simulink model "mintaveteles_FOXBORO_PI_szabalyozo"  (Simulink 8.7)
settings: Solver=VariableStepAuto  StartTime=0.0  StopTime=T_sim  RelTol=1e-3
values from neighbouring files (symbols this model uses):
  inv_u_stat = y_stat(i-1:end)    [Sebessegszabalyozas_sim.m]
  inv_y_stat = u_stat(i-1:end)    [Sebessegszabalyozas_sim.m]
  K = P1.Kp    [Sebessegszabalyozas_sim.m]
  K_C = 1/P1d.Numerator(2)*(1-exp(-Ts/T_cl))    [Sebessegszabalyozas_sim.m]
  P1d = c2d(sys,Ts,'zoh')    [Sebessegszabalyozas_sim.m]
  Ts = 0.01    [Sebessegszabalyozas_sim.m]
  u_sat = y_sat/K    [Sebessegszabalyozas_sim.m]
  u_stat = [0;100;200;250;300;350;400;450;500;550;600;700;750]    [Untitled.m]    (also in ident.mat = [0 100 200 300 400 500 600 700])
  y_stat = y_stat*K    [Sebessegszabalyozas_sim.m]    (also in Untitled.m = [0;  0;  0;  0; 42; 67; 80; 95;110;120;130;160;170]; ident.mat = [0 0 0 32 100 160 216 260])
  z_d = -P1d.Denominator(2)    [Sebessegszabalyozas_sim.m]
settings Model: Creator=Mester Ádám  LastModifiedBy=Mester Ádám
settings DataIOCC: LimitDataPoints=off  SaveFormat=Dataset
settings DebuggingCC: UnderspecifiedInitializationDetection=Simplified  MergeDetectMultiDrivingBlocksExec=error
settings HardwareCC: ProdBitPerPointer=64  ProdLargestAtomicFloat=Float  ProdIntDivRoundTo=Zero  ProdEndianess=LittleEndian  ProdWordSize=64  ProdHWDeviceType=Intel->x86-64 (Windows64)
settings ModelReferenceCC: PropagateSignalLabelsOutOfModel=on
settings ConfigComp: CovModelRefEnable=off

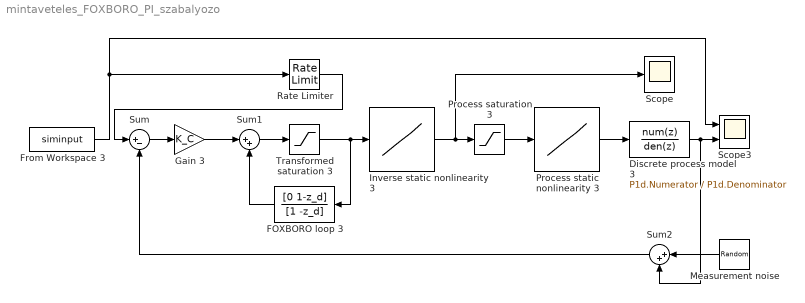
== system mintaveteles_FOXBORO_PI_szabalyozo ==
  Discrete process model 3 : DiscreteTransferFcn  Numerator=P1d.Numerator  Denominator=P1d.Denominator  SampleTime=Ts
  FOXBORO loop 3 : DiscreteTransferFcn  Numerator=[0 1-z_d]  Denominator=[1 -z_d]  SampleTime=Ts
  From Workspace 3 : FromWorkspace  VariableName=siminput  SampleTime=Ts
  Gain 3 : Gain  Gain=K_C
  Inverse static nonlinearity 3 : Lookup_n-D  NumberOfTableDimensions=1  BreakpointsForDimension1=inv_u_stat  Table=inv_y_stat  InternalRulePriority=Speed  RndMeth=Simplest  InputSameDT=on
  Measurement noise : RandomNumber  Variance=200*K  SampleTime=Ts
  Process saturation 3 : Saturate  UpperLimit=u_sat  LowerLimit=0
  Process static nonlinearity 3 : Lookup_n-D  NumberOfTableDimensions=1  BreakpointsForDimension1=u_stat  Table=y_stat  InternalRulePriority=Speed  RndMeth=Simplest  InputSameDT=on
  Rate Limiter : RateLimiter  RisingSlewLimit=3000*743/10000  FallingSlewLimit=-inf  SampleTimeMode=inherited
  Scope : Scope
  Scope3 : Scope  NumInputPorts=2
  Sum : Sum  Inputs=|+-
  Sum1 : Sum  Inputs=|++
  Sum2 : Sum  Inputs=|++
  Transformed saturation 3 : Saturate  UpperLimit=u_sat  LowerLimit=0
  wires:
  Discrete process model 3/1 -> Scope3/2, Sum2/2
  From Workspace 3/1 -> Rate Limiter/1, Scope3/1
  Process static nonlinearity 3/1 -> Discrete process model 3/1
  Process saturation 3/1 -> Process static nonlinearity 3/1
  Inverse static nonlinearity 3/1 -> Process saturation 3/1, Scope/1
  Sum/1 -> Gain 3/1
  Gain 3/1 -> Sum1/1
  Sum1/1 -> Transformed saturation 3/1
  FOXBORO loop 3/1 -> Sum1/2
  Measurement noise/1 -> Sum2/1
  Sum2/1 -> Sum/2
  Transformed saturation 3/1 -> FOXBORO loop 3/1, Inverse static nonlinearity 3/1
  Rate Limiter/1 -> Sum/1
